simulink model "ComplexRLCCircuit"  (R2020a)
settings: Solver=VariableStepAuto  StartTime=0.0  StopTime=50  RelTol=1e-3
settings Model: Creator=hp  LastModifiedBy=hp

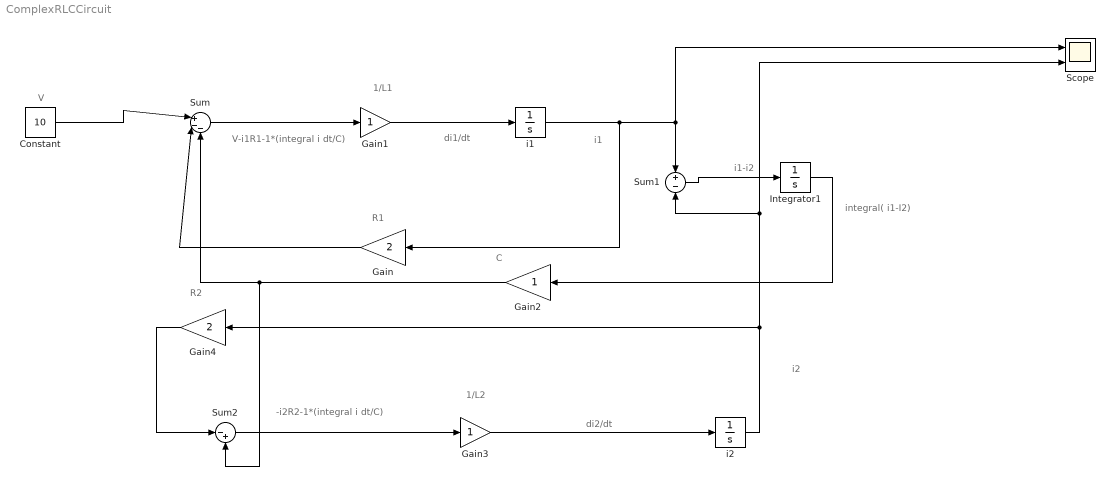
== system ComplexRLCCircuit ==
  note: integral( i1-I2)
  note: 1/L1
  note: V-i1R1-1*(integral i dt/C)
  note: V
  note: R1
  note: i1
  note: di2/dt
  note: di1/dt
  note: i2
  note: i1-i2
  note: C
  note: -i2R2-1*(integral i dt/C)
  note: R2
  note: 1/L2
  Constant : Constant  Value=10
  Gain : Gain  Gain=2
  Gain1 : Gain
  Gain2 : Gain
  Gain3 : Gain
  Gain4 : Gain  Gain=2
  Integrator1 : Integrator
  Scope : Scope  NumInputPorts=2
  Sum : Sum  Inputs=|+--
  Sum1 : Sum  Inputs=+-
  Sum2 : Sum  Inputs=|-+
  i1 : Integrator
  i2 : Integrator
  wires:
  Sum1/1 -> Integrator1/1
  Sum2/1 -> Gain3/1
  Gain4/1 -> Sum2/1
  Gain1/1 -> i1/1
  Gain2/1 -> Sum/3, Sum2/2
  Constant/1 -> Sum/1
  Sum/1 -> Gain1/1
  Gain/1 -> Sum/2
  Integrator1/1 -> Gain2/1
  i2/1 -> Scope/2, Sum1/2, Gain4/1
  i1/1 -> Scope/1, Sum1/1, Gain/1
  Gain3/1 -> i2/1
